simulink model "AI6109_MOA_AutoComp11"  (R2023b)
settings: Solver=FixedStepDiscrete  StartTime=0.0  StopTime=0.5  FixedStep=Ts  MaxStep=0.2  RelTol=1e-4  EnableMultiTasking=on
values from neighbouring files (symbols this model uses):
  f = figure('Color','w','Position',[100 100 1050 540])    [run_gating_ablation.m]    (also in run_m5_step5_robustness.m = context.dataF; run_phase2_simulink_dynamic.m = figure('Color','w','Position',[100 100 1000 520]))
undefined symbols (not defined in the file or in its folder): alpha_moa, C0, C_moa, Ccoupling_disabled_F, Cself_pF, h3_ratio, Iref_moa, phi3_deg, StopTime, Ts, Ts_model, Un_LL, Vneg_pu, Vref_moa
libraries: spsSeriesRLCBranchLib x13, spsCurrentMeasurementLib x6, spsVoltageMeasurementLib x6, spsGroundLib x4, spsControlledCurrentSourceLib x3, spsThreePhaseProgrammableVoltageSourceLib x1, spspowerguiLib x1
settings Model: Creator=18423  LastModifiedBy=18423
settings SolverCC: AlgebraicLoopSolver=TrustRegion  MaxZcPerStep=1
settings DataIOCC: LimitDataPoints=on  MaxDataPoints=10000  ReturnWorkspaceOutputs=off
settings OptimizationCC: ReuseModelBlockBuffer=off  LifeSpan=inf
settings DebuggingCC: UnconnectedInputMsg=warning  UnconnectedOutputMsg=warning  UnconnectedLineMsg=warning  AllowSymbolicDim=off  SFUnexpectedBacktrackingDiag=warning  SFNoUnconditionalDefaultTransitionDiag=warning  SFExecutionAtInitializationDiag=none  ArithmeticOperatorsInVariantConditions=warning
settings ModelReferenceCC: EnableRefExpFcnMdlSchedulingChecks=on
settings SFSimCC: SimUseLocalCustomCode=off  CustomCodeUndefinedFunction=UseInterfaceOnly
settings RTWCC: RTWUseLocalCustomCode=off  DLArmComputeVersion=19.05
settings CodeAppCC: StateflowObjectComments=on
settings GRTTargetCC: TargetLangStandard=C89/C90 (ANSI)
settings ConfigComp: CovMetricSettings=dw  CovSaveCumulativeToWorkspaceVar=on  CovSaveSingleToWorkspaceVar=on  CovExternalEMLEnable=off  CovSFcnEnable=off
settings SimscapeCC: SimscapeLogType=all  SimscapeLogDataHistory=10000

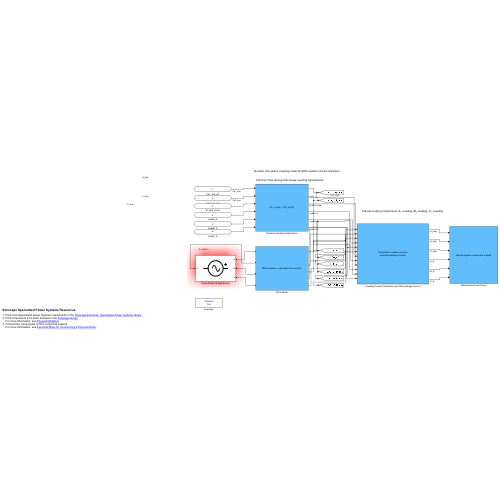
[thumbnail: Simulink's stored preview of the top-level diagram]
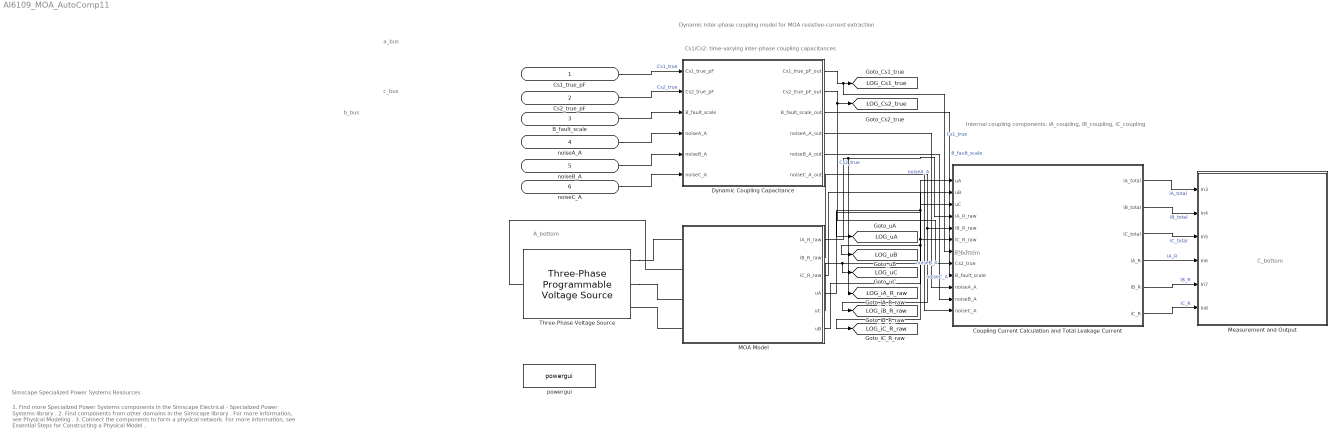
== system AI6109_MOA_AutoComp11 ==
  note: A_bottom
  note: c_bus
  note: b_bus
  note: a_bus
  note: 1. Find more Specialized Power Systems components in the Simscape Electrical - Specialized Power Systems library .
      | 2. Find components from other domains in the Simscape library .
      | For more information, see Physical Modeling .
      | 3. Connect the components to form a physical network.
      | For more information, see Essential Steps for Constructing a Physical Model .
  note: Simscape Specialized Power Systems Resources
  note: B_bottom
  note: C_bottom
  note: Dynamic inter-phase coupling model for MOA resistive-current extraction
  note: Cs1/Cs2: time-varying inter-phase coupling capacitances
  note: Internal coupling components: iA_coupling, iB_coupling, iC_coupling
  Cs1_true_pF : Inport
  Cs2_true_pF : Inport  Port=2
  B_fault_scale : Inport  Port=3
  noiseA_A : Inport  Port=4
  noiseB_A : Inport  Port=5
  noiseC_A : Inport  Port=6
  Coupling Current Calculation and Total Leakage Current : Subsystem
      mask Display: disp('Inter-phase coupling currents\nand total leakage currents');
  Dynamic Coupling Capacitance : Subsystem
      mask Display: disp('Cs1_true(t)   Cs2_true(t)');
  MOA Model : Subsystem
      mask Display: disp('MOA resistive + self-capacitive currents');
  Measurement and Output : Subsystem
      mask Display: disp('Named signals / workspace outputs');
  Three-Phase Voltage Source : spsThreePhaseProgrammableVoltageSourceLib/Three-Phase Programmable Voltage Source  PositiveSequence="[Un_LL  120 f]"  VariationEntity=None  VariationType=Table of time-amplitude pairs  VariationTypeAlt=Step  VariationStep=0.5  VariationRate=10  VariationMagnitude=0.3  VariationFrequency=2  VariationTiming=[1 2]  VariationPhaseA=off  Amplitudes=[1 0.8 1.2 1.0]  TimeValues=[0 0.1 0.15 0.2]  HarmonicGeneration=on  HarmonicA=[3 h3_ratio phi3_deg 0]  HarmonicB=[1 Vneg_pu 0 2]  Timing="[0  StopTime]"  BusType=swing  Pref=0  Qref=0  Qmin=-inf  Qmax=inf
  powergui : spspowerguiLib/powergui  Priority=1  SimulationMode=Discrete  SampleTime=Ts  frequency=60  Iterations=50  frequencyindice=50  Pbase=100e6  ErrMax=1e-4  UnitsV=kV  UnitsW=MW  buscounter=0  FunctionMessages=off  echomessages=off  EnableUseOfTLC=off  CurrentSourceSwitches=off  DisableSnubberDevices=off  DisableRonSwitches=off  DisableVfSwitches=off  DisplayEquations=off  AutomaticDiscreteSolvers=off  SolverType=Tustin/Backward Euler (TBE)  Interpol=off  ExternalGateDelay=off  methode=off  Ts=100  x0status=blocks  SPID=on  SwTol=0  HookPort=off  NonlinearTolerance=0  nMaxIteration=15  ContinueOnMaxIteration=off  RestoreLinks=warning  ResistiveCurrentMeasurement=off  Frange=[0:2:500]  Ylog=off  Xlog=on  ShowGrid=off  save=off  variable=ZData  structure=0  ZoomFFT=off  StartTime=0.0  cycles=1  DisplayStyle=1  fundamental=60  FreqAxis=off  MaxFrequency=1000  frequencyindicesteady=1  RmsSteady=1  display=off
  tag scope: LOG_Cs1_true=global, LOG_Cs2_true=global, LOG_iA_R_raw=global, LOG_iB_R_raw=global, LOG_iC_R_raw=global, LOG_uA=global, LOG_uB=global, LOG_uC=global
  wires:
  Cs1_true_pF/1 -> Dynamic Coupling Capacitance/1(Cs1_true_pF)  "Cs1_true"
  Dynamic Coupling Capacitance/1(Cs1_true_pF_out) -> Coupling Current Calculation and Total Leakage Current/7(Cs1_true), [LOG_Cs1_true]  "Cs1_true"
  Cs2_true_pF/1 -> Dynamic Coupling Capacitance/2(Cs2_true_pF)  "Cs2_true"
  Dynamic Coupling Capacitance/2(Cs2_true_pF_out) -> Coupling Current Calculation and Total Leakage Current/8(Cs2_true), [LOG_Cs2_true]  "Cs2_true"
  B_fault_scale/1 -> Dynamic Coupling Capacitance/3(B_fault_scale)
  noiseA_A/1 -> Dynamic Coupling Capacitance/4(noiseA_A)
  noiseB_A/1 -> Dynamic Coupling Capacitance/5(noiseB_A)
  noiseC_A/1 -> Dynamic Coupling Capacitance/6(noiseC_A)
  Dynamic Coupling Capacitance/3(B_fault_scale_out) -> Coupling Current Calculation and Total Leakage Current/9(B_fault_scale)  "B_fault_scale"
  Dynamic Coupling Capacitance/4(noiseA_A_out) -> Coupling Current Calculation and Total Leakage Current/10(noiseA_A)  "noiseA_A"
  Dynamic Coupling Capacitance/5(noiseB_A_out) -> Coupling Current Calculation and Total Leakage Current/11(noiseB_A)  "noiseB_A"
  Dynamic Coupling Capacitance/6(noiseC_A_out) -> Coupling Current Calculation and Total Leakage Current/12(noiseC_A)  "noiseC_A"
  Coupling Current Calculation and Total Leakage Current/1(iA_total) -> Measurement and Output/1(In3)  "iA_total"
  Coupling Current Calculation and Total Leakage Current/2(iB_total) -> Measurement and Output/2(In4)  "iB_total"
  Coupling Current Calculation and Total Leakage Current/3(iC_total) -> Measurement and Output/3(In5)  "iC_total"
  Coupling Current Calculation and Total Leakage Current/4(iA_R) -> Measurement and Output/4(In6)  "iA_R"
  Coupling Current Calculation and Total Leakage Current/5(iB_R) -> Measurement and Output/5(In7)  "iB_R"
  Coupling Current Calculation and Total Leakage Current/6(iC_R) -> Measurement and Output/6(In8)  "iC_R"
  MOA Model/2(iB_R_raw) -> [LOG_iB_R_raw], Coupling Current Calculation and Total Leakage Current/5(iB_R_raw)
  MOA Model/5(uC) -> Coupling Current Calculation and Total Leakage Current/3(uC), [LOG_uC]
  MOA Model/4(uA) -> [LOG_uA], Coupling Current Calculation and Total Leakage Current/1(uA)
  MOA Model/6(uB) -> [LOG_uB], Coupling Current Calculation and Total Leakage Current/2(uB)
  MOA Model/1(iA_R_raw) -> Coupling Current Calculation and Total Leakage Current/4(iA_R_raw), [LOG_iA_R_raw]
  MOA Model/3(iC_R_raw) -> [LOG_iC_R_raw], Coupling Current Calculation and Total Leakage Current/6(iC_R_raw)
  connections:
  Three-Phase Voltage Source/RConn1 -- MOA Model/LConn1
  MOA Model/LConn2 -- Three-Phase Voltage Source/LConn1
  Three-Phase Voltage Source/RConn2 -- MOA Model/LConn3
  MOA Model/LConn4 -- Three-Phase Voltage Source/RConn3

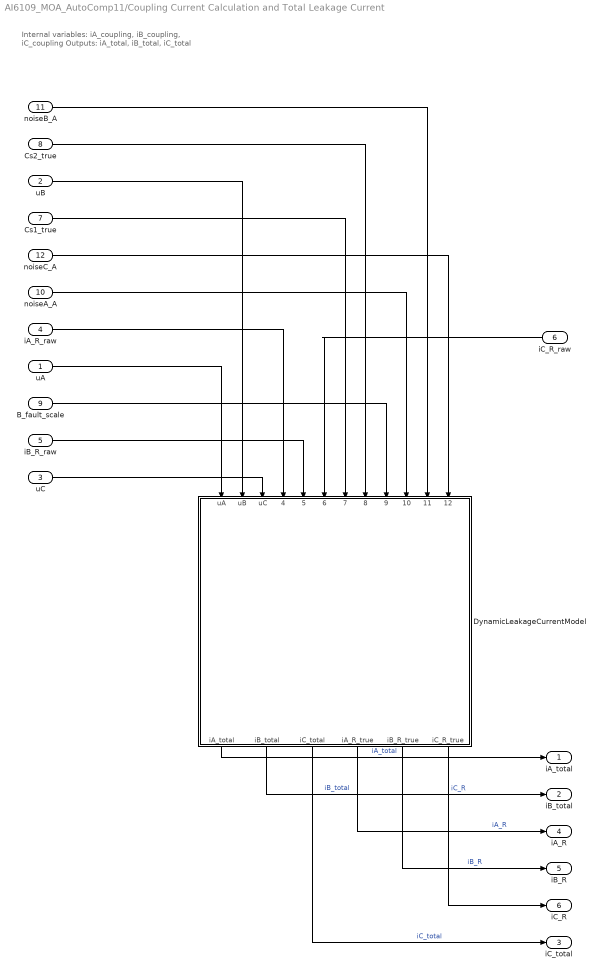
== system AI6109_MOA_AutoComp11/Coupling Current Calculation and Total Leakage Current ==
  note: Internal variables:
      | iA_coupling, iB_coupling, iC_coupling
      | Outputs: iA_total, iB_total, iC_total
  uA : Inport
  uB : Inport  Port=2
  uC : Inport  Port=3
  iA_R_raw : Inport  Port=4
  iB_R_raw : Inport  Port=5
  iC_R_raw : Inport  Port=6
  Cs1_true : Inport  Port=7
  Cs2_true : Inport  Port=8
  B_fault_scale : Inport  Port=9
  noiseA_A : Inport  Port=10
  noiseB_A : Inport  Port=11
  noiseC_A : Inport  Port=12
  DynamicLeakageCurrentModel : MATLAB Function  TreatAsAtomicUnit=on
  iA_total : Outport
  iB_total : Outport  Port=2
  iC_total : Outport  Port=3
  iA_R : Outport  Port=4
  iB_R : Outport  Port=5
  iC_R : Outport  Port=6
  wires:
  uA/1 -> DynamicLeakageCurrentModel/1(uA)
  noiseA_A/1 -> DynamicLeakageCurrentModel/10(noiseA)
  iA_R_raw/1 -> DynamicLeakageCurrentModel/4(iA_R_raw)
  Cs1_true/1 -> DynamicLeakageCurrentModel/7(Cs1_pF)
  noiseB_A/1 -> DynamicLeakageCurrentModel/11(noiseB)
  uB/1 -> DynamicLeakageCurrentModel/2(uB)
  Cs2_true/1 -> DynamicLeakageCurrentModel/8(Cs2_pF)
  noiseC_A/1 -> DynamicLeakageCurrentModel/12(noiseC)
  iC_R_raw/1 -> DynamicLeakageCurrentModel/6(iC_R_raw)
  B_fault_scale/1 -> DynamicLeakageCurrentModel/9(B_fault_scale)
  iB_R_raw/1 -> DynamicLeakageCurrentModel/5(iB_R_raw)
  uC/1 -> DynamicLeakageCurrentModel/3(uC)
  DynamicLeakageCurrentModel/6(iC_R_true) -> iC_R/1  "iC_R"
  DynamicLeakageCurrentModel/3(iC_total) -> iC_total/1  "iC_total"
  DynamicLeakageCurrentModel/5(iB_R_true) -> iB_R/1  "iB_R"
  DynamicLeakageCurrentModel/2(iB_total) -> iB_total/1  "iB_total"
  DynamicLeakageCurrentModel/4(iA_R_true) -> iA_R/1  "iA_R"
  DynamicLeakageCurrentModel/1(iA_total) -> iA_total/1  "iA_total"

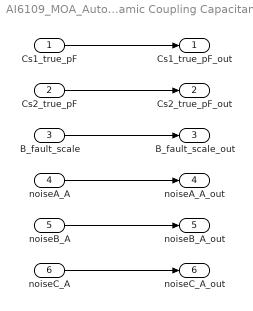
== system AI6109_MOA_AutoComp11/Dynamic Coupling Capacitance ==
  Cs1_true_pF : Inport
  Cs2_true_pF : Inport  Port=2
  B_fault_scale : Inport  Port=3
  noiseA_A : Inport  Port=4
  noiseB_A : Inport  Port=5
  noiseC_A : Inport  Port=6
  Cs1_true_pF_out : Outport
  Cs2_true_pF_out : Outport  Port=2
  B_fault_scale_out : Outport  Port=3
  noiseA_A_out : Outport  Port=4
  noiseB_A_out : Outport  Port=5
  noiseC_A_out : Outport  Port=6
  wires:
  Cs1_true_pF/1 -> Cs1_true_pF_out/1
  Cs2_true_pF/1 -> Cs2_true_pF_out/1
  B_fault_scale/1 -> B_fault_scale_out/1
  noiseA_A/1 -> noiseA_A_out/1
  noiseB_A/1 -> noiseB_A_out/1
  noiseC_A/1 -> noiseC_A_out/1

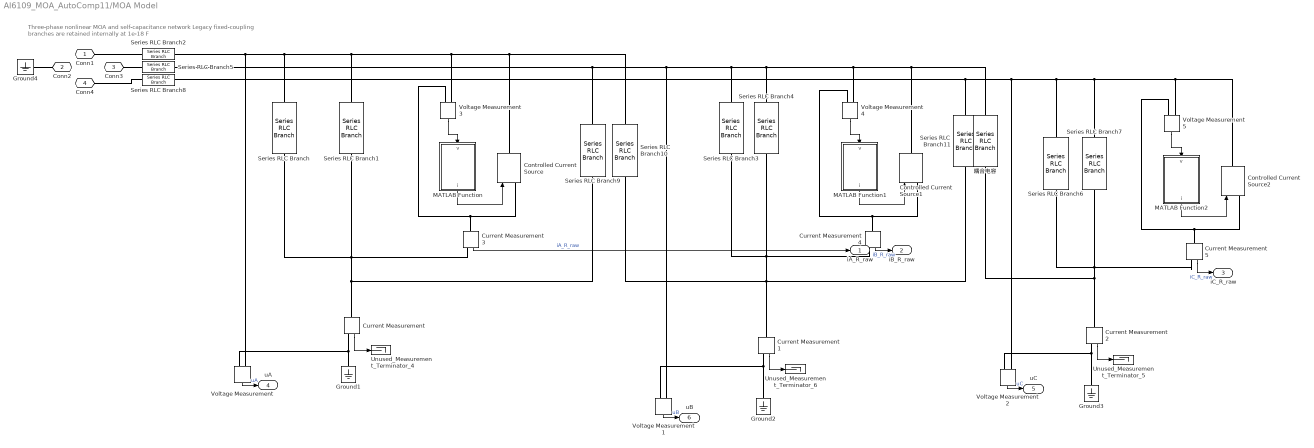
== system AI6109_MOA_AutoComp11/MOA Model ==
  note: Three-phase nonlinear MOA and self-capacitance network
      | Legacy fixed-coupling branches are retained internally at 1e-18 F
  Controlled Current Source : spsControlledCurrentSourceLib/Controlled Current Source  Initialize=on  Source_Type=AC  Amplitude=0  Phase=0  Frequency=0  Measurements=None
  Controlled Current Source1 : spsControlledCurrentSourceLib/Controlled Current Source  Initialize=on  Source_Type=AC  Amplitude=0  Phase=0  Frequency=0  Measurements=None
  Controlled Current Source2 : spsControlledCurrentSourceLib/Controlled Current Source  Initialize=on  Source_Type=AC  Amplitude=0  Phase=0  Frequency=0  Measurements=None
  Current Measurement{,1..5} (6 alike) : spsCurrentMeasurementLib/Current Measurement  PhasorSimulation=off  OutputType=Complex  PSBequivalent=0
  Ground{1..4} (4 alike) : spsGroundLib/Ground  LConnTagsString=a
  MATLAB Function : MATLAB Function  TreatAsAtomicUnit=on
  MATLAB Function1 : MATLAB Function  TreatAsAtomicUnit=on
  MATLAB Function2 : MATLAB Function  TreatAsAtomicUnit=on
  Series RLC Branch : spsSeriesRLCBranchLib/Series RLC Branch  LConnTagsString=__new0  RConnTagsString=__new0  BranchType=C  Resistance=1  Inductance=1e-3  SetiL0=off  InitialCurrent=0  Capacitance=C0  Setx0=off  InitialVoltage=0  Measurements=None
  Series RLC Branch1 : spsSeriesRLCBranchLib/Series RLC Branch  LConnTagsString=__new0  RConnTagsString=__new0  BranchType=C  Resistance=1  Inductance=1e-3  SetiL0=off  InitialCurrent=0  Capacitance=C_moa  Setx0=off  InitialVoltage=0  Measurements=None
  Series RLC Branch10 : spsSeriesRLCBranchLib/Series RLC Branch  LConnTagsString=__new0  RConnTagsString=__new0  BranchType=C  Resistance=1  Inductance=1e-3  SetiL0=off  InitialCurrent=0  Capacitance=Ccoupling_disabled_F  Setx0=off  InitialVoltage=0  Measurements=None
  Series RLC Branch11 : spsSeriesRLCBranchLib/Series RLC Branch  LConnTagsString=__new0  RConnTagsString=__new0  BranchType=C  Resistance=1  Inductance=1e-3  SetiL0=off  InitialCurrent=0  Capacitance=Ccoupling_disabled_F  Setx0=off  InitialVoltage=0  Measurements=None
  Series RLC Branch2 : spsSeriesRLCBranchLib/Series RLC Branch  LConnTagsString=__new0  RConnTagsString=__new0  BranchType=R  Resistance=0.1  Inductance=1e-3  SetiL0=off  InitialCurrent=0  Capacitance=C_moa  Setx0=off  InitialVoltage=0  Measurements=None
  Series RLC Branch3 : spsSeriesRLCBranchLib/Series RLC Branch  LConnTagsString=__new0  RConnTagsString=__new0  BranchType=C  Resistance=1  Inductance=1e-3  SetiL0=off  InitialCurrent=0  Capacitance=C0  Setx0=off  InitialVoltage=0  Measurements=None
  Series RLC Branch4 : spsSeriesRLCBranchLib/Series RLC Branch  LConnTagsString=__new0  RConnTagsString=__new0  BranchType=C  Resistance=1  Inductance=1e-3  SetiL0=off  InitialCurrent=0  Capacitance=C_moa  Setx0=off  InitialVoltage=0  Measurements=None
  Series RLC Branch5 : spsSeriesRLCBranchLib/Series RLC Branch  LConnTagsString=__new0  RConnTagsString=__new0  BranchType=R  Resistance=0.1  Inductance=1e-3  SetiL0=off  InitialCurrent=0  Capacitance=C_moa  Setx0=off  InitialVoltage=0  Measurements=None
  Series RLC Branch6 : spsSeriesRLCBranchLib/Series RLC Branch  LConnTagsString=__new0  RConnTagsString=__new0  BranchType=C  Resistance=1  Inductance=1e-3  SetiL0=off  InitialCurrent=0  Capacitance=C0  Setx0=off  InitialVoltage=0  Measurements=None
  Series RLC Branch7 : spsSeriesRLCBranchLib/Series RLC Branch  LConnTagsString=__new0  RConnTagsString=__new0  BranchType=C  Resistance=1  Inductance=1e-3  SetiL0=off  InitialCurrent=0  Capacitance=C_moa  Setx0=off  InitialVoltage=0  Measurements=None
  Series RLC Branch8 : spsSeriesRLCBranchLib/Series RLC Branch  LConnTagsString=__new0  RConnTagsString=__new0  BranchType=R  Resistance=0.1  Inductance=1e-3  SetiL0=off  InitialCurrent=0  Capacitance=C_moa  Setx0=off  InitialVoltage=0  Measurements=None
  Series RLC Branch9 : spsSeriesRLCBranchLib/Series RLC Branch  LConnTagsString=__new0  RConnTagsString=__new0  BranchType=C  Resistance=1  Inductance=1e-3  SetiL0=off  InitialCurrent=0  Capacitance=Ccoupling_disabled_F  Setx0=off  InitialVoltage=0  Measurements=None
  Unused_Measurement_Terminator_4 : Terminator
  Unused_Measurement_Terminator_5 : Terminator
  Unused_Measurement_Terminator_6 : Terminator
  Voltage Measurement{,1..5} (6 alike) : spsVoltageMeasurementLib/Voltage Measurement  PhasorSimulation=off  OutputType=Complex  PSBequivalent=0
  耦合电容 : spsSeriesRLCBranchLib/Series RLC Branch  LConnTagsString=__new0  RConnTagsString=__new0  BranchType=C  Resistance=1  Inductance=1e-3  SetiL0=off  InitialCurrent=0  Capacitance=Ccoupling_disabled_F  Setx0=off  InitialVoltage=0  Measurements=None
  Conn1 : PMIOPort  Side=Left
  Conn2 : PMIOPort  Port=2  Side=Left
  Conn3 : PMIOPort  Port=3  Side=Left
  Conn4 : PMIOPort  Port=4  Side=Left
  iA_R_raw : Outport
  iB_R_raw : Outport  Port=2
  iC_R_raw : Outport  Port=3
  uA : Outport  Port=4
  uC : Outport  Port=5
  uB : Outport  Port=6
  wires:
  Voltage Measurement3/1 -> MATLAB Function/1(v)
  MATLAB Function2/1(i) -> Controlled Current Source2/1
  MATLAB Function1/1(i) -> Controlled Current Source1/1
  Voltage Measurement4/1 -> MATLAB Function1/1(v)
  MATLAB Function/1(i) -> Controlled Current Source/1
  Voltage Measurement5/1 -> MATLAB Function2/1(v)
  Voltage Measurement1/1 -> uB/1  "uB"
  Voltage Measurement2/1 -> uC/1  "uC"
  Voltage Measurement/1 -> uA/1  "uA"
  Current Measurement4/1 -> iB_R_raw/1  "iB_R_raw"
  Current Measurement5/1 -> iC_R_raw/1  "iC_R_raw"
  Current Measurement3/1 -> iA_R_raw/1  "iA_R_raw"
  Current Measurement1/1 -> Unused_Measurement_Terminator_6/1
  Current Measurement2/1 -> Unused_Measurement_Terminator_5/1
  Current Measurement/1 -> Unused_Measurement_Terminator_4/1
  connections:
  Controlled Current Source1/LConn1 -- Current Measurement4/LConn1 -- Voltage Measurement4/LConn2
  Ground4/LConn1 -- Conn2/RConn1
  Controlled Current Source/RConn1 -- Series RLC Branch10/LConn1 -- Voltage Measurement3/LConn1 -- Series RLC Branch1/LConn1 -- Series RLC Branch2/RConn1 -- Voltage Measurement/LConn1 -- Series RLC Branch/LConn1
  Conn3/RConn1 -- Series RLC Branch5/LConn1
  Controlled Current Source2/LConn1 -- Current Measurement5/LConn1 -- Voltage Measurement5/LConn2
  Series RLC Branch/RConn1 -- Current Measurement3/RConn1 -- Series RLC Branch9/RConn1 -- Current Measurement/LConn1 -- Series RLC Branch1/RConn1
  Series RLC Branch11/LConn1 -- Series RLC Branch8/RConn1 -- Voltage Measurement2/LConn1 -- Voltage Measurement5/LConn1 -- Controlled Current Source2/RConn1 -- Series RLC Branch7/LConn1 -- Series RLC Branch6/LConn1
  Series RLC Branch3/RConn1 -- Series RLC Branch10/RConn1 -- Series RLC Branch11/RConn1 -- Current Measurement1/LConn1 -- Current Measurement4/RConn1 -- Series RLC Branch4/RConn1
  Ground2/LConn1 -- Voltage Measurement1/LConn2 -- Current Measurement1/RConn1
  Controlled Current Source/LConn1 -- Current Measurement3/LConn1 -- Voltage Measurement3/LConn2
  Series RLC Branch9/LConn1 -- Controlled Current Source1/RConn1 -- 耦合电容/LConn1 -- Voltage Measurement4/LConn1 -- Series RLC Branch4/LConn1 -- Series RLC Branch3/LConn1 -- Voltage Measurement1/LConn1 -- Series RLC Branch5/RConn1
  Series RLC Branch6/RConn1 -- Series RLC Branch7/RConn1 -- Current Measurement5/RConn1 -- Current Measurement2/LConn1 -- 耦合电容/RConn1
  Ground3/LConn1 -- Voltage Measurement2/LConn2 -- Current Measurement2/RConn1
  Ground1/LConn1 -- Current Measurement/RConn1 -- Voltage Measurement/LConn2
  Series RLC Branch8/LConn1 -- Conn4/RConn1
  Conn1/RConn1 -- Series RLC Branch2/LConn1

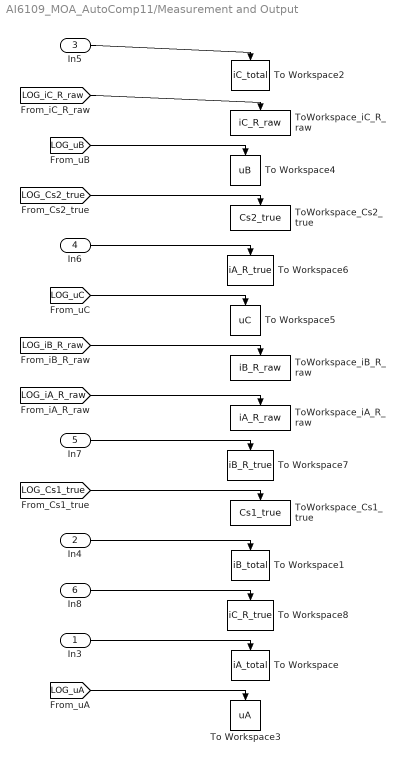
== system AI6109_MOA_AutoComp11/Measurement and Output ==
  In3 : Inport
  In4 : Inport  Port=2
  In5 : Inport  Port=3
  In6 : Inport  Port=4
  In7 : Inport  Port=5
  In8 : Inport  Port=6
  To Workspace : ToWorkspace  VariableName=iA_total  SaveFormat=Structure With Time  SampleTime=-1
  To Workspace1 : ToWorkspace  VariableName=iB_total  SaveFormat=Structure With Time  SampleTime=-1
  To Workspace2 : ToWorkspace  VariableName=iC_total  SaveFormat=Structure With Time  SampleTime=-1
  To Workspace3 : ToWorkspace  VariableName=uA  SaveFormat=Structure With Time  SampleTime=-1
  To Workspace4 : ToWorkspace  VariableName=uB  SaveFormat=Structure With Time  SampleTime=-1
  To Workspace5 : ToWorkspace  VariableName=uC  SaveFormat=Structure With Time  SampleTime=-1
  To Workspace6 : ToWorkspace  VariableName=iA_R_true  SaveFormat=Structure With Time  SampleTime=-1
  To Workspace7 : ToWorkspace  VariableName=iB_R_true  SaveFormat=Structure With Time  SampleTime=-1
  To Workspace8 : ToWorkspace  VariableName=iC_R_true  SaveFormat=Structure With Time  SampleTime=-1
  ToWorkspace_Cs1_true : ToWorkspace  VariableName=Cs1_true  SaveFormat=Structure With Time  SampleTime=-1
  ToWorkspace_Cs2_true : ToWorkspace  VariableName=Cs2_true  SaveFormat=Structure With Time  SampleTime=-1
  ToWorkspace_iA_R_raw : ToWorkspace  VariableName=iA_R_raw  SaveFormat=Structure With Time  SampleTime=-1
  ToWorkspace_iB_R_raw : ToWorkspace  VariableName=iB_R_raw  SaveFormat=Structure With Time  SampleTime=-1
  ToWorkspace_iC_R_raw : ToWorkspace  VariableName=iC_R_raw  SaveFormat=Structure With Time  SampleTime=-1
  wires:
  In6/1 -> To Workspace6/1
  In7/1 -> To Workspace7/1
  In5/1 -> To Workspace2/1
  [LOG_iB_R_raw] -> ToWorkspace_iB_R_raw/1
  [LOG_uC] -> To Workspace5/1
  [LOG_uB] -> To Workspace4/1
  [LOG_iC_R_raw] -> ToWorkspace_iC_R_raw/1
  [LOG_Cs2_true] -> ToWorkspace_Cs2_true/1
  [LOG_iA_R_raw] -> ToWorkspace_iA_R_raw/1
  [LOG_Cs1_true] -> ToWorkspace_Cs1_true/1
  In4/1 -> To Workspace1/1
  In8/1 -> To Workspace8/1
  In3/1 -> To Workspace/1
  [LOG_uA] -> To Workspace3/1

== matlab function AI6109_MOA_AutoComp11/MOA Model/MATLAB Function1 ==
  data: v input; i output; Vref_moa parameter; Iref_moa parameter; alpha_moa parameter
function i = moa_current(v, Vref_moa, Iref_moa, alpha_moa)
% 氧化锌避雷器非线性阻性电流模型（参数来自统一 cfg）
i = Iref_moa * sign(v) * (abs(v)/Vref_moa)^alpha_moa;
end

== matlab function AI6109_MOA_AutoComp11/MOA Model/MATLAB Function ==
  data: v input; i output; Vref_moa parameter; Iref_moa parameter; alpha_moa parameter
function i = moa_current(v, Vref_moa, Iref_moa, alpha_moa)
% 氧化锌避雷器非线性阻性电流模型（参数来自统一 cfg）
i = Iref_moa * sign(v) * (abs(v)/Vref_moa)^alpha_moa;
end

== matlab function AI6109_MOA_AutoComp11/MOA Model/MATLAB Function2 ==
  data: v input; i output; Vref_moa parameter; Iref_moa parameter; alpha_moa parameter
function i = moa_current(v, Vref_moa, Iref_moa, alpha_moa)
% 氧化锌避雷器非线性阻性电流模型（参数来自统一 cfg）
i = Iref_moa * sign(v) * (abs(v)/Vref_moa)^alpha_moa;
end

== matlab function AI6109_MOA_AutoComp11/Coupling Current Calculation and Total Leakage Current/DynamicLeakageCurrentModel ==
  data: uA input; uB input; uC input; iA_R_raw input; iA_total output; iB_R_raw input; iC_R_raw input; Cs1_pF input; Cs2_pF input; B_fault_scale input; noiseA input; noiseB input; noiseC input; iB_total output; iC_total output; iA_R_true output; iB_R_true output; iC_R_true output; Ts_model parameter; Cself_pF parameter
function [iA_total,iB_total,iC_total,iA_R_true,iB_R_true,iC_R_true] = dynamic_current(uA,uB, uC, iA_R_raw, iB_R_raw,iC_R_raw,Cs1_pF,Cs2_pF,B_fault_scale,noiseA,noiseB,noiseC, Ts_model, Cself_pF)
%#codegen
persistent a1 b1 c1 a2 b2 c2 count
if isempty(count), a1=uA; b1=uB; c1=uC; a2=uA; b2=uB; c2=uC; count=uint8(0); end
if count==0
 duA=0; duB=0; duC=0; count=uint8(1);
elseif count==1
 duA=(uA-a1)/Ts_model; duB=(uB-b1)/Ts_model; duC=(uC-c1)/Ts_model; count=uint8(2);
else
 duA=(3*uA-4*a1+a2)/(2*Ts_model); duB=(3*uB-4*b1+b2)/(2*Ts_model); duC=(3*uC-4*c1+c2)/(2*Ts_model);
end
a2=a1; b2=b1; c2=c1; a1=uA; b1=uB; c1=uC;
iA_R_true=-iA_R_raw; iB_R_true=-B_fault_scale*iB_R_raw; iC_R_true=-iC_R_raw;
Cs1=Cs1_pF*1e-12; Cs2=Cs2_pF*1e-12; Cself=Cself_pF*1e-12;
iA_total=Cself*duA+Cs1*(duA-duB)+iA_R_true+noiseA;
iB_total=Cself*duB+Cs1*(duB-duA)+Cs2*(duB-duC)+iB_R_true+noiseB;
iC_total=Cself*duC+Cs2*(duC-duB)+iC_R_true+noiseC;
end
